simulink library "reuse_lib"  (R2015b)
settings: Solver=ode45  StartTime=0.0  StopTime=10.0  RelTol=1e-3
settings Model: Creator=amatsumo  LastModifiedBy=amatsumo
settings DataIOCC: SaveFormat=Array
settings DebuggingCC: UnderspecifiedInitializationDetection=Classic  MergeDetectMultiDrivingBlocksExec=none  SolverPrmCheckMsg=warning
settings HardwareCC: ProdBitPerPointer=32  ProdLargestAtomicFloat=None  ProdIntDivRoundTo=Undefined  ProdEndianess=Unspecified  ProdWordSize=32  ProdHWDeviceType=32-bit Generic
settings GRTTargetCC: GeneratePreprocessorConditionals=Disable all
settings ConfigComp: CovModelRefEnable=Off  CovSFcnEnable=off

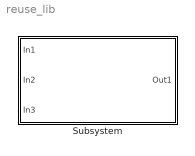
== system reuse_lib ==
  Subsystem : Subsystem  TreatAsAtomicUnit=on

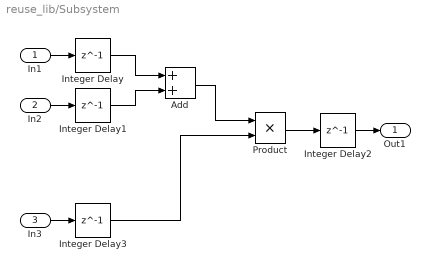
== system reuse_lib/Subsystem ==
  In1 : Inport
  In2 : Inport  Port=2
  In3 : Inport  Port=3
  Add : Sum
  Integer Delay{,1..3} (4 alike) : Delay  DelayLength=1  InputProcessing=Inherited
  Product : Product  RndMeth=Zero
  Out1 : Outport
  wires:
  In3/1 -> Integer Delay3/1
  Integer Delay2/1 -> Out1/1
  In2/1 -> Integer Delay1/1
  In1/1 -> Integer Delay/1
  Integer Delay3/1 -> Product/2
  Product/1 -> Integer Delay2/1
  Add/1 -> Product/1
  Integer Delay1/1 -> Add/2
  Integer Delay/1 -> Add/1
